simulink model "Trrafic_Light"  (R2021a)
settings: Solver=VariableStepAuto  StartTime=0.0  StopTime=10.0  RelTol=1e-3
settings Model: Creator=Moamen_Hamed  LastModifiedBy=Mahmoud Shams El-Din

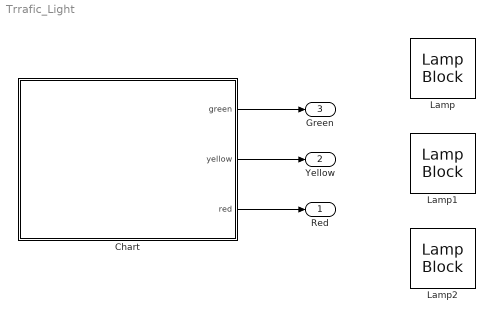
== system Trrafic_Light ==
  Chart : Stateflow chart  TreatAsAtomicUnit=on
  Lamp : LampBlock
  Lamp1 : LampBlock
  Lamp2 : LampBlock
  Red : Outport
  Yellow : Outport  Port=2
  Green : Outport  Port=3
  wires:
  Chart/3(red) -> Red/1
  Chart/2(yellow) -> Yellow/1
  Chart/1(green) -> Green/1

== stateflow chart Trrafic_Light/Chart ==
  state Red
    entry:
    red = 1;
    yellow = 0;
    green = 0;
  state Yellow
    entry:
    red = 0;
    yellow = 1;
    green = 0;
  state Green
    entry:
    red = 0;
    yellow = 0;
    green = 1;
  (default) -> Red
  Green -> Red : [after(1,sec)]
  Red -> Yellow : [after(1,sec)]
  Yellow -> Green : [after(1,sec)]
  data: green output; yellow output; red output
